simulink model "ODE_adsorption_Simulink"  (R2023a)
settings: Solver=FixedStepAuto  StartTime=0.0  StopTime=1500  FixedStep=0.001  RelTol=1e-3
values from neighbouring files (symbols this model uses):
  as = 6*(1-epsb)/dp    (= 600)    [ODE_adsorption_Generator.m]
  Cin = 1    [ODE_adsorption_Generator.m]
  epsb = 0.5    [ODE_adsorption_Generator.m]
  Ke = 10    [ODE_adsorption_Generator.m]
  kg = 0.0001    [ODE_adsorption_Generator.m]
  tau = 100    [ODE_adsorption_Generator.m]
settings Model: Creator=pierr  LastModifiedBy=pierr

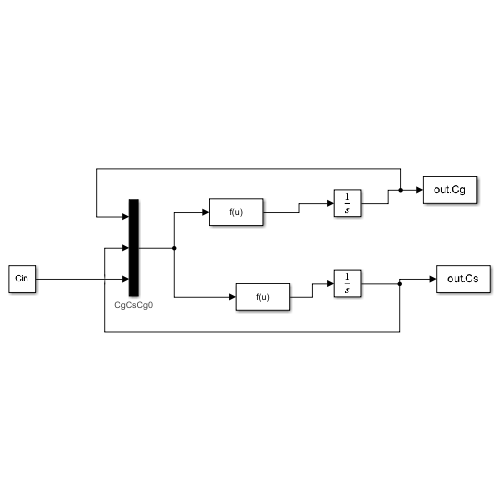
[thumbnail: Simulink's stored preview of the top-level diagram]
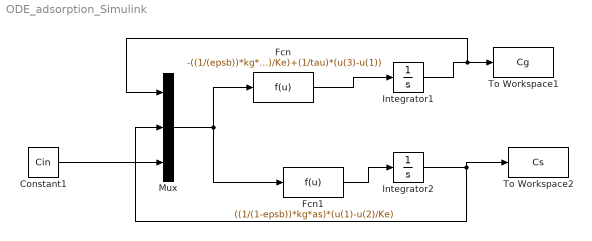
== system ODE_adsorption_Simulink ==
  Constant1 : Constant  Value=Cin
  Fcn : Fcn  Expr=-((1/(epsb))*kg*as)*(u(1)-u(2)/Ke)+(1/tau)*(u(3)-u(1))
  Fcn1 : Fcn  Expr=((1/(1-epsb))*kg*as)*(u(1)-u(2)/Ke)
  Integrator1 : Integrator
  Integrator2 : Integrator
  Mux : Mux  Inputs=3
      settings: AttributesFormatString=CgCsCg0
  To Workspace1 : ToWorkspace  VariableName=Cg  SaveFormat=Timeseries  SampleTime=-1
  To Workspace2 : ToWorkspace  VariableName=Cs  SaveFormat=Timeseries  SampleTime=-1
  wires:
  Integrator1/1 -> Mux/1, To Workspace1/1
  Fcn1/1 -> Integrator2/1
  Fcn/1 -> Integrator1/1
  Mux/1 -> Fcn1/1, Fcn/1
  Integrator2/1 -> To Workspace2/1, Mux/2
  Constant1/1 -> Mux/3
